simulink model "DigitalTwin_v8"  (R2023a)
settings: Solver=ode23t  StartTime=0.0  StopTime=600  RelTol=1e-3  AbsTol=1e-3
model workspace: external: MATLAB File C:\Users\claud\OneDrive - TUM\COME -TUM\Software lab\Three_wheeled_base\simscape_1\Three_wheeled_base_DataFile1.m (data not in the file)
values from neighbouring files (symbols this model uses):
  brick_pick_global_xy = [brick_pick_global_xy, new_column]    [Three_wheeled_base_DataFile2.m]
  brick_place_global_xy = [brick_place_global_xy, new_column]    [Three_wheeled_base_DataFile2.m]
  platform_destination_mat = [ 1.0 0; 5 0; 0 0; 0 5 ... (first row only)    [Three_wheeled_base_DataFile2.m]
  robotData =     [points_on_pad.mat]
  smiData =     [points_on_pad.mat]    (also in road_points_on_pad.mat)
undefined symbols (not defined in the file or in its folder): X, Y, Z
libraries: sm_lib x246, nesl_utility x86, fl_lib x12, batteryecm_lib x5, ee_lib x3, robotcorelib x1, robotalgslib x1
(part 8 of 8)

== matlab function DigitalTwin_v8/Task Scheduler ==
  data: platform_xy input; Theta_platform input; platformWaypoints output; platform_mode_out output; reset_time_out_arm output; arm_waypoints output; endtime_out output; arm_mode_out output; it_brick_out output; current_time input; brick_pick_relative input; brick_place_global_xy input; platform_destination_mat input; stop_simulation output
function [platformWaypoints,platform_mode_out, reset_time_out_arm,arm_waypoints, endtime_out,arm_mode_out, it_brick_out,stop_simulation] = task_scheduler(platform_xy,Theta_platform,current_time, brick_pick_relative, brick_place_global_xy, platform_destination_mat)

%-------------- Platform initialization  -----------------------------------------------------------------------

pickandplace_map = [2 4 6 8 10 12];
persistent previous_platform_position previous_platform_waypoints platform_destination
persistent  it_destination platform_move_begin platform_mode

if isempty(it_destination) 
    it_destination = 1;
    platform_destination = platform_destination_mat(1,:);
end

if isempty(platform_move_begin) 
    platform_move_begin = 1;
    platform_mode = 0;
end
if isempty(previous_platform_waypoints) 
    previous_platform_waypoints = zeros(2,2);
end
if isempty(previous_platform_position)
    previous_platform_position = zeros(1,2);
end

platformWaypoints=previous_platform_waypoints;

%-------------- End of platform initialization -----------------------------------------------------------------

%-------------- Arm initialization  -------------------------------------------------------------------------
brick_above = [0 0 0.4];
brick_grip_pos = [0 0 0.175];
persistent it_brick  arm_mode  reset_time_arm arm_move_finished previous_Arm_Waypoints total_Arm_Waypoints end_time 
if isempty(it_brick)
    it_brick = 1 ;
end
if isempty(previous_Arm_Waypoints) 
    previous_Arm_Waypoints = zeros(8,2);
    total_Arm_Waypoints = zeros(8,9);
end
if isempty(arm_mode) 
    arm_mode = 0;
    end_time = 3;
end
if isempty(reset_time_arm) 
    reset_time_arm = 0;
end
if isempty(arm_move_finished)
    arm_move_finished = 1 ;
end
coder.extrinsic("sm_kinovaGen3_arm_ik");
eeIgs = zeros(1,7);
%-------------- End of arm initialization -------------------------------------------------------------------

%-------------- Platform TS  -----------------------------------------------------------------------
distanceToRun = norm(platform_destination - platform_xy');


if platform_move_begin == 1 && (arm_mode == 0 || (arm_mode == 6 && current_time - reset_time_arm > end_time + 0.1 ) || (arm_mode == 11 && current_time - reset_time_arm > end_time + 0.1 ) ) && it_destination <= size(platform_destination_mat,1)
    disp("Entered platform scheduler")

    platform_move_begin = 0;
    platform_mode = 1;
    
    if  ismember(pickandplace_map(it_destination), pickandplace_map(1:2:end)) 
        platformWaypoints(1,:) = platform_destination_mat(pickandplace_map(it_destination)-1,:);
        platformWaypoints(2,:) = platform_destination_mat(pickandplace_map(it_destination)  ,:);
        platform_destination = platformWaypoints(2,:);

        
        distanceToRun = norm(platform_destination - platform_xy');
        disp("Mobile base started towards brick picking location at time: ")
        disp(current_time)
        disp("Platform waypoints are: ")
        disp(platformWaypoints)
        disp("Platform destination is")
        disp(platform_destination)

    elseif ismember (pickandplace_map(it_destination), pickandplace_map(2:2:end) )
        platformWaypoints(1,:) = platform_destination_mat(pickandplace_map(it_destination)-1,:);
        platformWaypoints(2,:) = platform_destination_mat(pickandplace_map(it_destination)  ,:);
        platform_destination = platformWaypoints(2,:);

        disp("Platform destination is")
        disp(platform_destination)
        distanceToRun = norm(platform_destination - platform_xy');
        disp("Mobile base started after picked brick at time: ")
        disp(current_time)
        disp("Platform waypoints are: ")
        disp(platformWaypoints)
        disp("Platform destination is")
        disp(platform_destination)

    end  

    if size(platform_destination_mat,1) >= it_destination
            it_destination = it_destination + 1;
    end

    previous_platform_waypoints = platformWaypoints;
    previous_platform_position = platform_destination;

end


if (platform_mode == 1) && distanceToRun<=0.01 
    disp("Mobile base movement finished at time")
    disp(current_time)
    disp("Mobile base origin is at ")
    disp(platform_xy)
    platform_mode = 0 ;
    if arm_mode == 0 || arm_mode == 11
        arm_mode = 1 ;
        previous_Arm_Waypoints = zeros(8,2);
        reset_time_arm =  current_time;
        end_time = 3;
    elseif arm_mode == 6
        arm_mode = 7 ;
    end        

end
%-------------- End of platform TS  -----------------------------------------------------------------------

%-------------- Arm TS  -----------------------------------------------------------------------
if it_brick <=3
relative_pick_pos = zeros(1,3);
relative_place_pos = zeros(1,3);
x_unrotated =  (brick_pick_relative(it_brick,1) );
y_unrotated =  (brick_pick_relative(it_brick,2) );
relative_pick_pos(1) =  x_unrotated * cos(-Theta_platform) - y_unrotated * sin(-Theta_platform) ;
relative_pick_pos(2) =  x_unrotated * sin(-Theta_platform) + y_unrotated * cos(-Theta_platform) ;
relative_pick_pos(3) = -0.033;
relative_place_pos(2) =  (brick_place_global_xy(it_brick,1) - platform_xy(1));
relative_place_pos(1) =  (brick_place_global_xy(it_brick,2) - platform_xy(2));
relative_place_pos(3) = brick_place_global_xy(it_brick,3);
else
    arm_mode = 12; 
    relative_place_pos = zeros(1,3);
    relative_pick_pos = zeros(1,3);
end

% relative_pick_pos(1) =  (brick_pick_global_xy(it_brick,1) - platform_xy(1));
% relative_pick_pos(2) =  (brick_pick_global_xy(it_brick,2) - platform_xy(2));
% relative_pick_pos(3) = -0.033;
% x_unrotated =  (brick_place_global_xy(it_brick,1) - platform_xy(1));
% y_unrotated =  (brick_place_global_xy(it_brick,2) - platform_xy(2));
% relative_place_pos(1) =  x_unrotated * cos( pi/2 - Theta_platform) - y_unrotated * sin( pi/2 - Theta_platform) ;
% relative_place_pos(2) =  x_unrotated * sin( pi/2 - Theta_platform) + y_unrotated * cos( pi/2 - Theta_platform) ;
% relative_place_pos(3) = -0.03;

if arm_mode == 1  && current_time - reset_time_arm > end_time + 0.1
    arm_mode = 2 ;
    disp("Arm started approaching to pick at time")
    disp(current_time)
    disp("Brick is located wrt arm origin is")
    disp(relative_pick_pos)

    TR_frame = [
    [relative_pick_pos+brick_above,[180 0 Theta_platform*(180/pi)]];...
    [relative_pick_pos+brick_grip_pos,[180 0 Theta_platform*(180/pi)]];...
    [relative_pick_pos+brick_grip_pos,[180 0 Theta_platform*(180/pi)]];...
    [relative_pick_pos+brick_above,[180 0 Theta_platform*(180/pi)]] ];...
    % [relative_place_pos+brick_grip_pos,[180 0 0]];...
    % [relative_place_pos+brick_grip_pos,[180 0 0]];...
    % [relative_place_pos+brick_above,[180 0 0]]];
    [solution,solvedFlag] =  sm_kinovaGen3_arm_ik(TR_frame,eeIgs);
    total_Arm_Waypoints(1:7,:) = [zeros(7,1) solution zeros(7,4)];
    total_Arm_Waypoints(1:7,2:size(TR_frame,1)+1) = total_Arm_Waypoints(1:7,2:size(TR_frame,1)+1)./180*pi;
    total_Arm_Waypoints(8,1:3)=0.0;
    total_Arm_Waypoints(8,4:5)= 0.4;

    previous_Arm_Waypoints = total_Arm_Waypoints(:,1:2);
    reset_time_arm = current_time ;
    end_time = 5;
elseif arm_mode == 2 && current_time - reset_time_arm > end_time + 0.1
    disp("Arm started going down to pick at time")
    disp(current_time)
    arm_mode = 3;
  
    previous_Arm_Waypoints(:,1) = previous_Arm_Waypoints(:,2);
    previous_Arm_Waypoints(:,2) = total_Arm_Waypoints(:,3);
    reset_time_arm = current_time ;
    end_time = 2.0;
elseif arm_mode == 3 && current_time - reset_time_arm > end_time + 0.1
    disp("Arm started closing grips to pick at time")
    disp(current_time)
    arm_mode = 4;
    previous_Arm_Waypoints(:,1) = previous_Arm_Waypoints(:,2);
    previous_Arm_Waypoints(:,2) = total_Arm_Waypoints(:,4);
    reset_time_arm = current_time ;
    end_time = 1.0;
elseif arm_mode == 4 && current_time - reset_time_arm > end_time + 0.1
    arm_mode = 5;
    disp("Arm picked and the gripper started moving a bit higher")
    disp(current_time)
    previous_Arm_Waypoints(:,1) = previous_Arm_Waypoints(:,2);
    previous_Arm_Waypoints(:,2) = total_Arm_Waypoints(:,5);

    reset_time_arm = current_time ;
    end_time = 2.0;
elseif arm_mode == 5 && current_time - reset_time_arm > end_time + 0.1
    disp("Arm start moving to the highest position")
    disp(current_time)
    arm_mode = 6;
    platform_move_begin = 1;
    previous_Arm_Waypoints(:,1) = previous_Arm_Waypoints(:,2);
    previous_Arm_Waypoints(1:7,2) = zeros(7,1);
    reset_time_arm = current_time ;
    end_time = 5.0;
elseif arm_mode == 7 && current_time  - reset_time_arm > end_time + 0.1
    arm_mode = 8;
    disp("Arm started approaching to place the brick at time")
    disp(current_time)
    disp("Place that brick will be placed wrt arm origin is ")
    disp(relative_place_pos)     
    
    TR_frame = [
    % [relative_pick_pos+brick_above,[180 0 0]];...
    % [relative_pick_pos+brick_grip_pos,[180 0 0]];...
    % [relative_pick_pos+brick_grip_pos,[180 0 0]];...
    % [relative_pick_pos+brick_above,[180 0 0]] ];...
    [relative_place_pos+brick_grip_pos, [180 0 Theta_platform*(180/pi)-90]];...
    [relative_place_pos+brick_grip_pos, [180 0 Theta_platform*(180/pi)-90]];...
    [relative_place_pos+brick_above,    [180 0 Theta_platform*(180/pi)-90]]];
    [solution] =  sm_kinovaGen3_arm_ik(TR_frame,eeIgs);
    total_Arm_Waypoints(1:7,6:8) = solution./180*pi; 
    total_Arm_Waypoints(8,6)= 0.2;
    total_Arm_Waypoints(8,7:8) = -0.3;
    previous_Arm_Waypoints(:,1) = previous_Arm_Waypoints(:,2);
    previous_Arm_Waypoints(:,2) = total_Arm_Waypoints(:,6);
    reset_time_arm = current_time ;
    end_time = 5.0;
 elseif arm_mode == 8 && current_time - reset_time_arm > end_time + 0.1
    disp("Arm opened grips")
    disp(current_time)
    arm_mode = 9;
    previous_Arm_Waypoints(:,1) = previous_Arm_Waypoints(:,2);
    previous_Arm_Waypoints(:,2) = total_Arm_Waypoints(:,7);
    reset_time_arm = current_time ;
    end_time = 1.0;
  elseif arm_mode == 9 && current_time - reset_time_arm > end_time + 0.1
    disp("Arm went upper after it left the brick")
    disp(current_time)
    arm_mode = 10;
    previous_Arm_Waypoints(:,1) = previous_Arm_Waypoints(:,2);
    previous_Arm_Waypoints(:,2) = total_Arm_Waypoints(:,8);
    reset_time_arm = current_time ;
    end_time = 2.0;
  elseif arm_mode == 10 && current_time - reset_time_arm > end_time + 0.1
    disp("Arm went initial position")
    disp(current_time)
    platform_move_begin = 1;
    arm_mode = 11;
    previous_Arm_Waypoints(:,1) = previous_Arm_Waypoints(:,2);
    previous_Arm_Waypoints(:,2) = total_Arm_Waypoints(:,9);
    reset_time_arm = current_time ;
    end_time = 5;
    it_brick = it_brick + 1;
end

if arm_mode >= 5 && arm_mode <= 8
    WS_switch = 0;
else
    WS_switch = -1;
end

arm_mode_out = arm_mode;
it_brick_out = it_brick;

reset_time_out_arm = reset_time_arm ;
arm_waypoints = previous_Arm_Waypoints;
endtime_out = end_time;
platform_mode_out = platform_mode;
stop_simulation = 0;

if arm_mode ==12 && current_time - reset_time_arm > end_time + 0.1
    stop_simulation = 1;
end
%-------------- End of TS  --------------------------------------------------------------------

end

== matlab function DigitalTwin_v8/Subsystem/Control/MATLAB Function ==
  data: goal_wL output; goal_wR output; xy input; target_position input; platform_mode_out input; velocity input; ang_vel input; distanceToRun output; velocity_out output
function [goal_wL, goal_wR, distanceToRun,velocity_out] = wheelVelocity(xy,target_position,platform_mode_out, velocity, ang_vel)
    wheelRadius=0.08;
    slowThreshold= 2;  %Distance to target where velocity should be reduced
    stopThreshold=0.1; %Target reached
    trackWidth=0.6124;
    stop = 0;
    % Slow the robot down when it's near the threshold
    distanceToRun = norm(target_position(end, :) - xy');
    % persistent trig_time slowmove_beg
    % if isempty(trig_time)
    %     trig_time = 0;
    %     slowmove_beg = 1;
    % end
    %Wheel speed computation
        %Slow base when it is close to the target
    distance_to_stop = 5*0.25/2;
    if distanceToRun <= distance_to_stop %%(distanceToRun<slowThreshold)
        velocity = sqrt(velocity^2 + (0-velocity)/(5)*2*(distance_to_stop -  distanceToRun)) ;
    end
    %Convert velocity to angular velocity in the wheels
    if platform_mode_out == 0  %%(distanceToRun<slowThreshold)
        velocity = 0;
        stop = 1;
        
    end

    velocity_out = velocity;
    goal_wL = +((velocity - trackWidth/2*ang_vel)/wheelRadius)*25/23*(1-stop);
    goal_wR = -((velocity + trackWidth/2*ang_vel)/wheelRadius)*25/23*(1-stop);
end

== matlab function DigitalTwin_v8/Subsystem/Control/MATLAB Function1 ==
  settings: updateMethod=DISCRETE
  data: goal_wL output; goal_wR output; xy input; target_position input; velocity input; ang_vel input; distanceToRun output; current_time input; velocity_out output
function [goal_wL, goal_wR, distanceToRun,velocity_out] = wheelVelocity(xy,target_position,velocity, ang_vel, current_time)
    wheelRadius=0.06;
    slowThreshold= 2;  %Distance to target where velocity should be reduced
    stopThreshold=0.1; %Target reached
    trackWidth=0.0925;
    stop = 1;
    % Slow the robot down when it's near the threshold
    distanceToRun = norm(target_position(end, :) - xy');
    persistent trig_time slowmove_beg
    if isempty(trig_time)
        trig_time = 0;
        slowmove_beg = 1;
    end
    %Wheel speed computation
        %Slow base when it is close to the target
    if (distanceToRun<slowThreshold)
        if slowmove_beg == 1
            slowmove_beg = 0;
            trig_time = current_time;
        end
        velocity= 0.1 - (0.1 / 4)*(current_time - trig_time);
            %Stop base when it is in the target area
        if (distanceToRun<=stopThreshold)
            slowmove_beg = 1;
            stop = 0;
        end
    end
        %Convert velocity to angular velocity in the wheels
    velocity_out = velocity;
    goal_wL = +((velocity - trackWidth/2*ang_vel)/wheelRadius)*stop;
    goal_wR = -((velocity + trackWidth/2*ang_vel)/wheelRadius)*stop;
end

== matlab function DigitalTwin_v8/Arm/Kinova Gen3 Arm/MATLAB Function ==
  data: arm_mode input; mode1 output; brick_iterator input; mode2 output; mode3 output
function [mode1,mode2,mode3]= fcn(arm_mode,brick_iterator)
mode1 = -1;
mode2 = -1;
mode3 = -1;
if arm_mode >= 5 && arm_mode <= 9 
    if brick_iterator == 1
        mode1 = 0;
    elseif brick_iterator == 2
        mode2 = 0;
    elseif brick_iterator == 3
        mode3 = 0;
    end
    
end
end
